simulink model "Vcu"  (R2020a)
settings: Solver=FixedStepDiscrete  StartTime=0.0  StopTime=10.0  FixedStep=ModelSimTime  RelTol=1e-3
PostLoadFcn:
  | , if any(exist('dsrtsu_mdlpostloadfcn', 'file') ~= 0), dsrtsu_mdlpostloadfcn('Execute', bdroot); end,
InitFcn:
  | , if any(exist('rtifpga_mdlclblib', 'file') ~= 0), rtifpga_mdlclblib('Init', bdroot); end,
undefined symbols (not defined in the file): rticanmm_blockfcn, rticanmm_initfcn, sigbuilder_block
libraries: rtimmsu_dsrtlib x5, commutil2 x1
(part 3 of 3)

== system Vcu/Controls /Signal Builder5 ==
  Demux : Demux  Tag=STV Demux  Outputs=1
      settings: DisplayOption=none
  FromWs : FromWorkspace  Tag=STV FromWs  VariableName=tuvar
      SigBuilderData=|
      | common.afterFinalStr = 'Extrapolate'
      | common.sampleTime = 0
      | dataSet.timeRange = [0 10]
      | dataSet.name = 'Group 1'
      | sbobj.Groups.Name = 'Group 1'
      | sbobj.Groups.Signals.Name = 'Driver Button'
      | sbobj.Groups.Signals.XData = [0 6 6 10]
      | sbobj.Groups.Signals.YData = [1 1 2 2]
  Driver Button : Outport  Tag=STV Outport  VectorParamsAs1DForOutWhenUnconnected=off
  wires:
  Demux/1 -> Driver Button/1
  FromWs/1 -> Demux/1

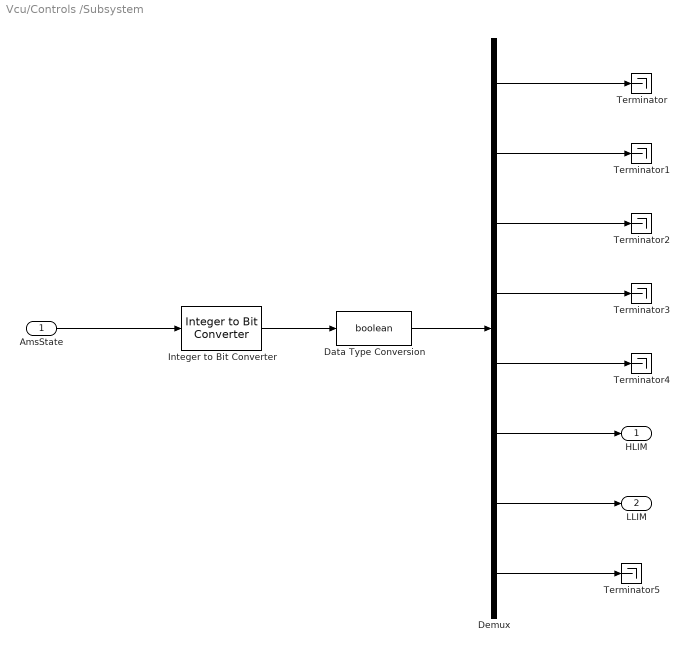
== system Vcu/Controls /Subsystem ==
  AmsState : Inport
  Data Type Conversion : DataTypeConversion  OutDataTypeStr=boolean
  Demux : Demux  Outputs=8
  Integer to Bit Converter : commutil2/Integer to Bit Converter  nbits=8  signedInputValues=Unsigned  bitOrder=LSB first  outDtype=Inherit via internal rule
  Terminator{,1..5} (6 alike) : Terminator
  HLIM : Outport  VectorParamsAs1DForOutWhenUnconnected=off
  LLIM : Outport  Port=2  VectorParamsAs1DForOutWhenUnconnected=off
  wires:
  Integer to Bit Converter/1 -> Data Type Conversion/1
  AmsState/1 -> Integer to Bit Converter/1
  Data Type Conversion/1 -> Demux/1
  Demux/1 -> Terminator/1
  Demux/2 -> Terminator1/1
  Demux/3 -> Terminator2/1
  Demux/4 -> Terminator3/1
  Demux/5 -> Terminator4/1
  Demux/7 -> LLIM/1
  Demux/6 -> HLIM/1
  Demux/8 -> Terminator5/1

== system Vcu/Controls /Triggering2RTICANMM MainBlock ==
  AMK0_ActualValues1 : Subsystem
  AMK0_ActualValues2 : Subsystem
  AMK0_SetPoints1 : Subsystem
  AMK1_ActualValues1 : Subsystem
  AMK1_ActualValues2 : Subsystem
  AMK1_SetPoints1 : Subsystem
  buscreator : BusCreator  Inputs=6
  out : Outport  VectorParamsAs1DForOutWhenUnconnected=off
  wires:
  AMK0_ActualValues1/1(out) -> buscreator/1  "AMK0_ActualValues1"
  AMK0_ActualValues2/1(out) -> buscreator/2  "AMK0_ActualValues2"
  AMK0_SetPoints1/1(out) -> buscreator/3  "AMK0_SetPoints1"
  AMK1_ActualValues1/1(out) -> buscreator/4  "AMK1_ActualValues1"
  AMK1_ActualValues2/1(out) -> buscreator/5  "AMK1_ActualValues2"
  AMK1_SetPoints1/1(out) -> buscreator/6  "AMK1_SetPoints1"
  buscreator/1 -> out/1  "CAN"

== system Vcu/Controls /User2RTICANMM MainBlock ==
  in : Inport
  AMK0_SetPoints1 : Subsystem
  AMK1_SetPoints1 : Subsystem
  buscreator : BusCreator  Inputs=2
  out : Outport  VectorParamsAs1DForOutWhenUnconnected=off
  wires:
  AMK0_SetPoints1/1(out) -> buscreator/1  "AMK0_SetPoints1"
  AMK1_SetPoints1/1(out) -> buscreator/2  "AMK1_SetPoints1"
  in/1 -> AMK0_SetPoints1/1(in), AMK1_SetPoints1/1(in)
  buscreator/1 -> out/1  "CAN"

== system Vcu/Controls /User2RTICANMM MainBlock1 ==
  in : Inport
  AMK0_SetPoints1 : Subsystem
  AMK1_SetPoints1 : Subsystem
  buscreator : BusCreator  Inputs=2
  out : Outport  VectorParamsAs1DForOutWhenUnconnected=off
  wires:
  AMK0_SetPoints1/1(out) -> buscreator/1  "AMK0_SetPoints1"
  AMK1_SetPoints1/1(out) -> buscreator/2  "AMK1_SetPoints1"
  in/1 -> AMK0_SetPoints1/1(in), AMK1_SetPoints1/1(in)
  buscreator/1 -> out/1  "CAN"

== system Vcu/Controls /User2RTICANMM MainBlock2 ==
  CoolingLoopModes : Subsystem
  TemperatureInfo : Subsystem
  VehicleInfo : Subsystem
  buscreator : BusCreator  Inputs=3
  out : Outport  VectorParamsAs1DForOutWhenUnconnected=off
  wires:
  CoolingLoopModes/1(out) -> buscreator/1  "CoolingLoopModes"
  TemperatureInfo/1(out) -> buscreator/2  "TemperatureInfo"
  VehicleInfo/1(out) -> buscreator/3  "VehicleInfo"
  buscreator/1 -> out/1  "CAN"

== system Vcu/Controls /User2RTICANMM MainBlock3 ==
  in : Inport
  ELP_ContactorRequest : Subsystem
  buscreator : BusCreator  Inputs=1
  out : Outport  VectorParamsAs1DForOutWhenUnconnected=off
  wires:
  ELP_ContactorRequest/1(out) -> buscreator/1  "ELP_ContactorRequest"
  in/1 -> ELP_ContactorRequest/1(in)
  buscreator/1 -> out/1  "CAN"

== system Vcu/RTICANMM ControllerSetup/ModelClose ==

== system Vcu/RTICANMM ControllerSetup1/ModelClose ==

== system Vcu/RTICANMM ControllerSetup2/ModelClose ==

== system Vcu/RTICANMM ControllerSetup3/ModelClose ==

== system Vcu/RTICANMM GeneralSetup/ModelClose ==

== system Vcu/Controls /RTICANMM MainBlock/ModelClose ==

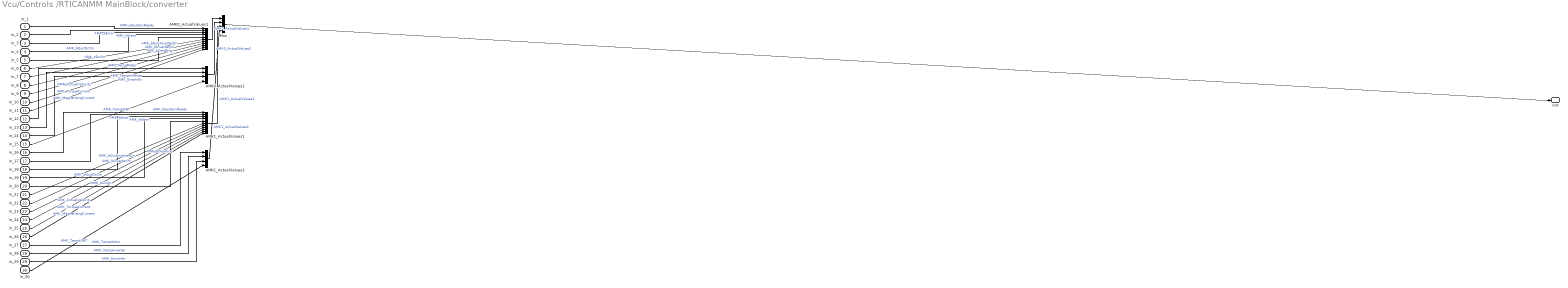
== system Vcu/Controls /RTICANMM MainBlock/converter ==
  in_1 : Inport
  in_2 : Inport  Port=2
  in_3 : Inport  Port=3
  in_4 : Inport  Port=4
  in_5 : Inport  Port=5
  in_6 : Inport  Port=6
  in_7 : Inport  Port=7
  in_8 : Inport  Port=8
  in_9 : Inport  Port=9
  in_10 : Inport  Port=10
  in_11 : Inport  Port=11
  in_12 : Inport  Port=12
  in_13 : Inport  Port=13
  in_14 : Inport  Port=14
  in_15 : Inport  Port=15
  in_16 : Inport  Port=16
  in_17 : Inport  Port=17
  in_18 : Inport  Port=18
  in_19 : Inport  Port=19
  in_20 : Inport  Port=20
  in_21 : Inport  Port=21
  in_22 : Inport  Port=22
  in_23 : Inport  Port=23
  in_24 : Inport  Port=24
  in_25 : Inport  Port=25
  in_26 : Inport  Port=26
  in_27 : Inport  Port=27
  in_28 : Inport  Port=28
  in_29 : Inport  Port=29
  in_30 : Inport  Port=30
  AMK0_ActualValues1 : BusCreator  Inputs=11
  AMK0_ActualValues2 : BusCreator  Inputs=4
  AMK1_ActualValues1 : BusCreator  Inputs=11
  AMK1_ActualValues2 : BusCreator  Inputs=4
  Mux : BusCreator  Inputs=4
  out : Outport
  wires:
  in_1/1 -> AMK0_ActualValues1/1  "AMK_bSystemReady"
  AMK0_ActualValues1/1 -> Mux/1  "AMK0_ActualValues1"
  in_2/1 -> AMK0_ActualValues1/2  "AMK_bError"
  in_3/1 -> AMK0_ActualValues1/3  "AMK_bWarn"
  in_4/1 -> AMK0_ActualValues1/4  "AMK_bQuitDcOn"
  in_5/1 -> AMK0_ActualValues1/5  "AMK_bDcOn"
  in_6/1 -> AMK0_ActualValues1/6  "AMK_bQuitInverterOn"
  in_7/1 -> AMK0_ActualValues1/7  "AMK_bInverterOn"
  in_8/1 -> AMK0_ActualValues1/8  "AMK_bDerating"
  in_9/1 -> AMK0_ActualValues1/9  "AMK_ActualVelocity"
  in_10/1 -> AMK0_ActualValues1/10  "AMK_TorqueCurrent"
  in_11/1 -> AMK0_ActualValues1/11  "AMK_MagnetizingCurrent"
  in_12/1 -> AMK0_ActualValues2/1  "AMK_TempMotor"
  AMK0_ActualValues2/1 -> Mux/2  "AMK0_ActualValues2"
  in_13/1 -> AMK0_ActualValues2/2  "AMK_TempInverter"
  in_14/1 -> AMK0_ActualValues2/3  "AMK_ErrorInfo"
  in_15/1 -> AMK0_ActualValues2/4  "AMK_TempIGBT"
  in_16/1 -> AMK1_ActualValues1/1  "AMK_bSystemReady"
  AMK1_ActualValues1/1 -> Mux/3  "AMK1_ActualValues1"
  in_17/1 -> AMK1_ActualValues1/2  "AMK_bError"
  in_18/1 -> AMK1_ActualValues1/3  "AMK_bWarn"
  in_19/1 -> AMK1_ActualValues1/4  "AMK_bQuitDcOn"
  in_20/1 -> AMK1_ActualValues1/5  "AMK_bDcOn"
  in_21/1 -> AMK1_ActualValues1/6  "AMK_bQuitInverterOn"
  in_22/1 -> AMK1_ActualValues1/7  "AMK_bInverterOn"
  in_23/1 -> AMK1_ActualValues1/8  "AMK_bDerating"
  in_24/1 -> AMK1_ActualValues1/9  "AMK_ActualVelocity"
  in_25/1 -> AMK1_ActualValues1/10  "AMK_TorqueCurrent"
  in_26/1 -> AMK1_ActualValues1/11  "AMK_MagnetizingCurrent"
  in_27/1 -> AMK1_ActualValues2/1  "AMK_TempMotor"
  AMK1_ActualValues2/1 -> Mux/4  "AMK1_ActualValues2"
  in_28/1 -> AMK1_ActualValues2/2  "AMK_TempInverter"
  in_29/1 -> AMK1_ActualValues2/3  "AMK_ErrorInfo"
  in_30/1 -> AMK1_ActualValues2/4  "AMK_TempIGBT"
  Mux/1 -> out/1

== system Vcu/Controls /RTICANMM MainBlock1/ModelClose ==

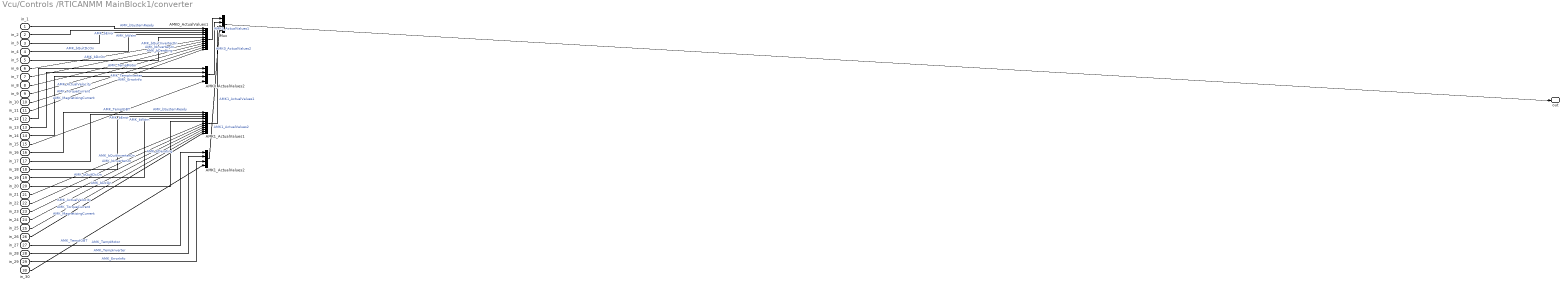
== system Vcu/Controls /RTICANMM MainBlock1/converter ==
  in_1 : Inport
  in_2 : Inport  Port=2
  in_3 : Inport  Port=3
  in_4 : Inport  Port=4
  in_5 : Inport  Port=5
  in_6 : Inport  Port=6
  in_7 : Inport  Port=7
  in_8 : Inport  Port=8
  in_9 : Inport  Port=9
  in_10 : Inport  Port=10
  in_11 : Inport  Port=11
  in_12 : Inport  Port=12
  in_13 : Inport  Port=13
  in_14 : Inport  Port=14
  in_15 : Inport  Port=15
  in_16 : Inport  Port=16
  in_17 : Inport  Port=17
  in_18 : Inport  Port=18
  in_19 : Inport  Port=19
  in_20 : Inport  Port=20
  in_21 : Inport  Port=21
  in_22 : Inport  Port=22
  in_23 : Inport  Port=23
  in_24 : Inport  Port=24
  in_25 : Inport  Port=25
  in_26 : Inport  Port=26
  in_27 : Inport  Port=27
  in_28 : Inport  Port=28
  in_29 : Inport  Port=29
  in_30 : Inport  Port=30
  AMK0_ActualValues1 : BusCreator  Inputs=11
  AMK0_ActualValues2 : BusCreator  Inputs=4
  AMK1_ActualValues1 : BusCreator  Inputs=11
  AMK1_ActualValues2 : BusCreator  Inputs=4
  Mux : BusCreator  Inputs=4
  out : Outport
  wires:
  in_1/1 -> AMK0_ActualValues1/1  "AMK_bSystemReady"
  AMK0_ActualValues1/1 -> Mux/1  "AMK0_ActualValues1"
  in_2/1 -> AMK0_ActualValues1/2  "AMK_bError"
  in_3/1 -> AMK0_ActualValues1/3  "AMK_bWarn"
  in_4/1 -> AMK0_ActualValues1/4  "AMK_bQuitDcOn"
  in_5/1 -> AMK0_ActualValues1/5  "AMK_bDcOn"
  in_6/1 -> AMK0_ActualValues1/6  "AMK_bQuitInverterOn"
  in_7/1 -> AMK0_ActualValues1/7  "AMK_bInverterOn"
  in_8/1 -> AMK0_ActualValues1/8  "AMK_bDerating"
  in_9/1 -> AMK0_ActualValues1/9  "AMK_ActualVelocity"
  in_10/1 -> AMK0_ActualValues1/10  "AMK_TorqueCurrent"
  in_11/1 -> AMK0_ActualValues1/11  "AMK_MagnetizingCurrent"
  in_12/1 -> AMK0_ActualValues2/1  "AMK_TempMotor"
  AMK0_ActualValues2/1 -> Mux/2  "AMK0_ActualValues2"
  in_13/1 -> AMK0_ActualValues2/2  "AMK_TempInverter"
  in_14/1 -> AMK0_ActualValues2/3  "AMK_ErrorInfo"
  in_15/1 -> AMK0_ActualValues2/4  "AMK_TempIGBT"
  in_16/1 -> AMK1_ActualValues1/1  "AMK_bSystemReady"
  AMK1_ActualValues1/1 -> Mux/3  "AMK1_ActualValues1"
  in_17/1 -> AMK1_ActualValues1/2  "AMK_bError"
  in_18/1 -> AMK1_ActualValues1/3  "AMK_bWarn"
  in_19/1 -> AMK1_ActualValues1/4  "AMK_bQuitDcOn"
  in_20/1 -> AMK1_ActualValues1/5  "AMK_bDcOn"
  in_21/1 -> AMK1_ActualValues1/6  "AMK_bQuitInverterOn"
  in_22/1 -> AMK1_ActualValues1/7  "AMK_bInverterOn"
  in_23/1 -> AMK1_ActualValues1/8  "AMK_bDerating"
  in_24/1 -> AMK1_ActualValues1/9  "AMK_ActualVelocity"
  in_25/1 -> AMK1_ActualValues1/10  "AMK_TorqueCurrent"
  in_26/1 -> AMK1_ActualValues1/11  "AMK_MagnetizingCurrent"
  in_27/1 -> AMK1_ActualValues2/1  "AMK_TempMotor"
  AMK1_ActualValues2/1 -> Mux/4  "AMK1_ActualValues2"
  in_28/1 -> AMK1_ActualValues2/2  "AMK_TempInverter"
  in_29/1 -> AMK1_ActualValues2/3  "AMK_ErrorInfo"
  in_30/1 -> AMK1_ActualValues2/4  "AMK_TempIGBT"
  Mux/1 -> out/1

== system Vcu/Controls /RTICANMM MainBlock2/ModelClose ==

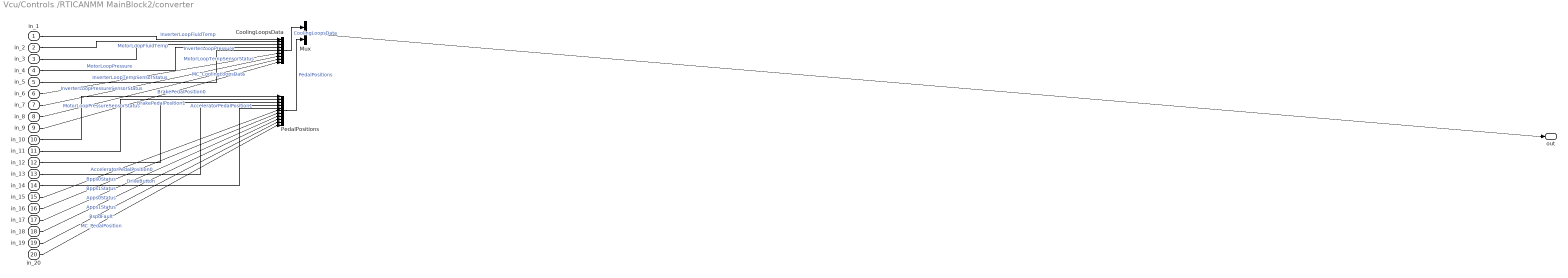
== system Vcu/Controls /RTICANMM MainBlock2/converter ==
  in_1 : Inport
  in_2 : Inport  Port=2
  in_3 : Inport  Port=3
  in_4 : Inport  Port=4
  in_5 : Inport  Port=5
  in_6 : Inport  Port=6
  in_7 : Inport  Port=7
  in_8 : Inport  Port=8
  in_9 : Inport  Port=9
  in_10 : Inport  Port=10
  in_11 : Inport  Port=11
  in_12 : Inport  Port=12
  in_13 : Inport  Port=13
  in_14 : Inport  Port=14
  in_15 : Inport  Port=15
  in_16 : Inport  Port=16
  in_17 : Inport  Port=17
  in_18 : Inport  Port=18
  in_19 : Inport  Port=19
  in_20 : Inport  Port=20
  CoolingLoopsData : BusCreator  Inputs=9
  Mux : BusCreator  Inputs=2
  PedalPositions : BusCreator  Inputs=11
  out : Outport
  wires:
  in_1/1 -> CoolingLoopsData/1  "InverterLoopFluidTemp"
  CoolingLoopsData/1 -> Mux/1  "CoolingLoopsData"
  in_2/1 -> CoolingLoopsData/2  "MotorLoopFluidTemp"
  in_3/1 -> CoolingLoopsData/3  "InverterLoopPressure"
  in_4/1 -> CoolingLoopsData/4  "MotorLoopPressure"
  in_5/1 -> CoolingLoopsData/5  "InverterLoopTempSensorStatus"
  in_6/1 -> CoolingLoopsData/6  "MotorLoopTempSensorStatus"
  in_7/1 -> CoolingLoopsData/7  "InverterLoopPressureSensorStatus"
  in_8/1 -> CoolingLoopsData/8  "MotorLoopPressureSensorStatus"
  in_9/1 -> CoolingLoopsData/9  "MC_CoolingLoopsData"
  in_10/1 -> PedalPositions/1  "BrakePedalPosition0"
  PedalPositions/1 -> Mux/2  "PedalPositions"
  in_11/1 -> PedalPositions/2  "BrakePedalPosition1"
  in_12/1 -> PedalPositions/3  "AcceleratorPedalPosition1"
  in_13/1 -> PedalPositions/4  "AcceleratorPedalPosition0"
  in_14/1 -> PedalPositions/5  "DriveButton"
  in_15/1 -> PedalPositions/6  "Bpps0Status"
  in_16/1 -> PedalPositions/7  "Bpps1Status"
  in_17/1 -> PedalPositions/8  "Apps0Status"
  in_18/1 -> PedalPositions/9  "Apps1Status"
  in_19/1 -> PedalPositions/10  "BspdFault"
  in_20/1 -> PedalPositions/11  "MC_PedalPosition"
  Mux/1 -> out/1

== system Vcu/Controls /RTICANMM MainBlock3/ModelClose ==

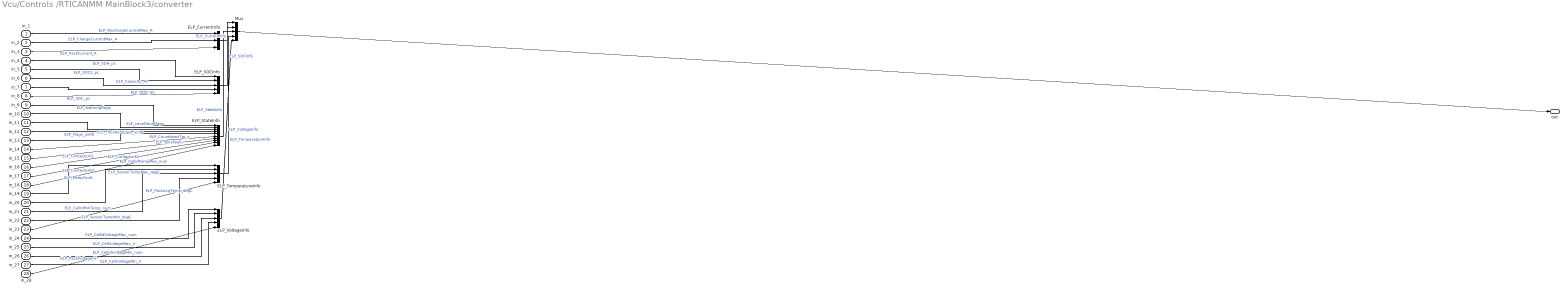
== system Vcu/Controls /RTICANMM MainBlock3/converter ==
  in_1 : Inport
  in_2 : Inport  Port=2
  in_3 : Inport  Port=3
  in_4 : Inport  Port=4
  in_5 : Inport  Port=5
  in_6 : Inport  Port=6
  in_7 : Inport  Port=7
  in_8 : Inport  Port=8
  in_9 : Inport  Port=9
  in_10 : Inport  Port=10
  in_11 : Inport  Port=11
  in_12 : Inport  Port=12
  in_13 : Inport  Port=13
  in_14 : Inport  Port=14
  in_15 : Inport  Port=15
  in_16 : Inport  Port=16
  in_17 : Inport  Port=17
  in_18 : Inport  Port=18
  in_19 : Inport  Port=19
  in_20 : Inport  Port=20
  in_21 : Inport  Port=21
  in_22 : Inport  Port=22
  in_23 : Inport  Port=23
  in_24 : Inport  Port=24
  in_25 : Inport  Port=25
  in_26 : Inport  Port=26
  in_27 : Inport  Port=27
  in_28 : Inport  Port=28
  ELP_CurrentInfo : BusCreator  Inputs=3
  ELP_SOCInfo : BusCreator  Inputs=5
  ELP_StateInfo : BusCreator  Inputs=10
  ELP_TemperatureInfo : BusCreator  Inputs=5
  ELP_VoltageInfo : BusCreator  Inputs=5
  Mux : BusCreator  Inputs=5
  out : Outport
  wires:
  in_1/1 -> ELP_CurrentInfo/1  "ELP_DischargeCurrentMax_A"
  ELP_CurrentInfo/1 -> Mux/1  "ELP_CurrentInfo"
  in_2/1 -> ELP_CurrentInfo/2  "ELP_ChargeCurrentMax_A"
  in_3/1 -> ELP_CurrentInfo/3  "ELP_PackCurrent_A"
  in_4/1 -> ELP_SOCInfo/1  "ELP_SOH_pc"
  ELP_SOCInfo/1 -> Mux/2  "ELP_SOCInfo"
  in_5/1 -> ELP_SOCInfo/2  "ELP_SOC2_pc"
  in_6/1 -> ELP_SOCInfo/3  "ELP_Capacity_Ah"
  in_7/1 -> ELP_SOCInfo/4  "ELP_DOD_Ah"
  in_8/1 -> ELP_SOCInfo/5  "ELP_SOC_pc"
  in_9/1 -> ELP_StateInfo/1  "ELP_WarningFlags"
  ELP_StateInfo/1 -> Mux/3  "ELP_StateInfo"
  in_10/1 -> ELP_StateInfo/2  "ELP_LevelFaultFlags"
  in_11/1 -> ELP_StateInfo/3  "ELP_FltCodeStored_uint8"
  in_12/1 -> ELP_StateInfo/4  "ELP_Flags_uint8"
  in_13/1 -> ELP_StateInfo/5  "ELP_CountdownTm_s"
  in_14/1 -> ELP_StateInfo/6  "ELP_BmsFault"
  in_15/1 -> ELP_StateInfo/7  "ELP_ContactorK1"
  in_16/1 -> ELP_StateInfo/8  "ELP_ContactorK2"
  in_17/1 -> ELP_StateInfo/9  "ELP_ContactorK3"
  in_18/1 -> ELP_StateInfo/10  "ELP_RelayFault"
  in_19/1 -> ELP_TemperatureInfo/1  "ELP_CellIdTempMax_num"
  ELP_TemperatureInfo/1 -> Mux/4  "ELP_TemperatureInfo"
  in_20/1 -> ELP_TemperatureInfo/2  "ELP_SensorTempMax_degC"
  in_21/1 -> ELP_TemperatureInfo/3  "ELP_CellIdMinTemp_num"
  in_22/1 -> ELP_TemperatureInfo/4  "ELP_SensorTempMin_degC"
  in_23/1 -> ELP_TemperatureInfo/5  "ELP_PackAvgTemp_degC"
  in_24/1 -> ELP_VoltageInfo/1  "ELP_CellIdVoltageMax_num"
  ELP_VoltageInfo/1 -> Mux/5  "ELP_VoltageInfo"
  in_25/1 -> ELP_VoltageInfo/2  "ELP_CellVoltageMax_V"
  in_26/1 -> ELP_VoltageInfo/3  "ELP_CellIdVoltageMin_num"
  in_27/1 -> ELP_VoltageInfo/4  "ELP_CellVoltageMin_V"
  in_28/1 -> ELP_VoltageInfo/5  "ELP_PackVoltage_V"
  Mux/1 -> out/1

== system Vcu/Controls /Triggering2RTICANMM MainBlock/AMK0_ActualValues1 ==
  AMK0_ActualValues1_CycleTime : Constant  Value=0
  buscreator : BusCreator  Inputs=1
  dt_AMK0_ActualValues1_CycleTime : DataTypeConversion  RndMeth=Zero
  out : Outport
  wires:
  buscreator/1 -> out/1  "AMK0_ActualValues1"
  AMK0_ActualValues1_CycleTime/1 -> dt_AMK0_ActualValues1_CycleTime/1
  dt_AMK0_ActualValues1_CycleTime/1 -> buscreator/1  "AMK0_ActualValues1_CycleTime"

== system Vcu/Controls /Triggering2RTICANMM MainBlock/AMK0_ActualValues2 ==
  AMK0_ActualValues2_CycleTime : Constant  Value=0
  buscreator : BusCreator  Inputs=1
  dt_AMK0_ActualValues2_CycleTime : DataTypeConversion  RndMeth=Zero
  out : Outport
  wires:
  buscreator/1 -> out/1  "AMK0_ActualValues2"
  AMK0_ActualValues2_CycleTime/1 -> dt_AMK0_ActualValues2_CycleTime/1
  dt_AMK0_ActualValues2_CycleTime/1 -> buscreator/1  "AMK0_ActualValues2_CycleTime"

== system Vcu/Controls /Triggering2RTICANMM MainBlock/AMK0_SetPoints1 ==
  AMK0_SetPoints1_CycleTime : Constant  Value=0
  buscreator : BusCreator  Inputs=1
  dt_AMK0_SetPoints1_CycleTime : DataTypeConversion  RndMeth=Zero
  out : Outport
  wires:
  buscreator/1 -> out/1  "AMK0_SetPoints1"
  AMK0_SetPoints1_CycleTime/1 -> dt_AMK0_SetPoints1_CycleTime/1
  dt_AMK0_SetPoints1_CycleTime/1 -> buscreator/1  "AMK0_SetPoints1_CycleTime"

== system Vcu/Controls /Triggering2RTICANMM MainBlock/AMK1_ActualValues1 ==
  AMK1_ActualValues1_CycleTime : Constant  Value=0
  buscreator : BusCreator  Inputs=1
  dt_AMK1_ActualValues1_CycleTime : DataTypeConversion  RndMeth=Zero
  out : Outport
  wires:
  buscreator/1 -> out/1  "AMK1_ActualValues1"
  AMK1_ActualValues1_CycleTime/1 -> dt_AMK1_ActualValues1_CycleTime/1
  dt_AMK1_ActualValues1_CycleTime/1 -> buscreator/1  "AMK1_ActualValues1_CycleTime"

== system Vcu/Controls /Triggering2RTICANMM MainBlock/AMK1_ActualValues2 ==
  AMK1_ActualValues2_CycleTime : Constant  Value=0
  buscreator : BusCreator  Inputs=1
  dt_AMK1_ActualValues2_CycleTime : DataTypeConversion  RndMeth=Zero
  out : Outport
  wires:
  buscreator/1 -> out/1  "AMK1_ActualValues2"
  AMK1_ActualValues2_CycleTime/1 -> dt_AMK1_ActualValues2_CycleTime/1
  dt_AMK1_ActualValues2_CycleTime/1 -> buscreator/1  "AMK1_ActualValues2_CycleTime"

== system Vcu/Controls /Triggering2RTICANMM MainBlock/AMK1_SetPoints1 ==
  AMK1_SetPoints1_CycleTime : Constant  Value=0
  buscreator : BusCreator  Inputs=1
  dt_AMK1_SetPoints1_CycleTime : DataTypeConversion  RndMeth=Zero
  out : Outport
  wires:
  buscreator/1 -> out/1  "AMK1_SetPoints1"
  AMK1_SetPoints1_CycleTime/1 -> dt_AMK1_SetPoints1_CycleTime/1
  dt_AMK1_SetPoints1_CycleTime/1 -> buscreator/1  "AMK1_SetPoints1_CycleTime"

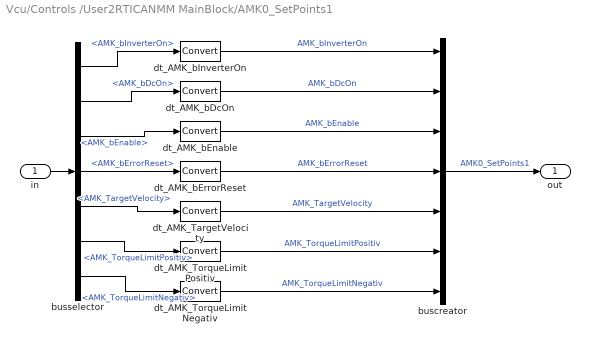
== system Vcu/Controls /User2RTICANMM MainBlock/AMK0_SetPoints1 ==
  in : Inport
  buscreator : BusCreator  Inputs=7
  busselector : BusSelector  OutputSignals=Inverter1FL.AMK_bInverterOn,Inverter1FL.AMK_bDcOn,Inverter1FL.AMK_bEnable,Inverter1FL.AMK_bErrorReset,Inverter1FL.AMK_TargetVelocity,Inverter1FL.AMK_TorqueLimitPositiv,Inverter1FL.AMK_TorqueLimitNegativ
  dt_AMK_TargetVelocity : DataTypeConversion  RndMeth=Zero
  dt_AMK_TorqueLimitNegativ : DataTypeConversion  RndMeth=Zero
  dt_AMK_TorqueLimitPositiv : DataTypeConversion  RndMeth=Zero
  dt_AMK_bDcOn : DataTypeConversion  RndMeth=Zero
  dt_AMK_bEnable : DataTypeConversion  RndMeth=Zero
  dt_AMK_bErrorReset : DataTypeConversion  RndMeth=Zero
  dt_AMK_bInverterOn : DataTypeConversion  RndMeth=Zero
  out : Outport
  wires:
  buscreator/1 -> out/1  "AMK0_SetPoints1"
  in/1 -> busselector/1
  busselector/1 -> dt_AMK_bInverterOn/1  "<AMK_bInverterOn>"
  dt_AMK_bInverterOn/1 -> buscreator/1  "AMK_bInverterOn"
  busselector/2 -> dt_AMK_bDcOn/1  "<AMK_bDcOn>"
  dt_AMK_bDcOn/1 -> buscreator/2  "AMK_bDcOn"
  busselector/3 -> dt_AMK_bEnable/1  "<AMK_bEnable>"
  dt_AMK_bEnable/1 -> buscreator/3  "AMK_bEnable"
  busselector/4 -> dt_AMK_bErrorReset/1  "<AMK_bErrorReset>"
  dt_AMK_bErrorReset/1 -> buscreator/4  "AMK_bErrorReset"
  busselector/5 -> dt_AMK_TargetVelocity/1  "<AMK_TargetVelocity>"
  dt_AMK_TargetVelocity/1 -> buscreator/5  "AMK_TargetVelocity"
  busselector/6 -> dt_AMK_TorqueLimitPositiv/1  "<AMK_TorqueLimitPositiv>"
  dt_AMK_TorqueLimitPositiv/1 -> buscreator/6  "AMK_TorqueLimitPositiv"
  busselector/7 -> dt_AMK_TorqueLimitNegativ/1  "<AMK_TorqueLimitNegativ>"
  dt_AMK_TorqueLimitNegativ/1 -> buscreator/7  "AMK_TorqueLimitNegativ"

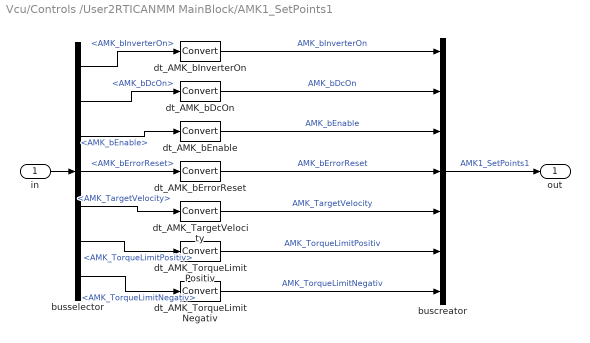
== system Vcu/Controls /User2RTICANMM MainBlock/AMK1_SetPoints1 ==
  in : Inport
  buscreator : BusCreator  Inputs=7
  busselector : BusSelector  OutputSignals=Inverter2FR.AMK_bInverterOn,Inverter2FR.AMK_bDcOn,Inverter2FR.AMK_bEnable,Inverter2FR.AMK_bErrorReset,Inverter2FR.AMK_TargetVelocity,Inverter2FR.AMK_TorqueLimitPositiv,Inverter2FR.AMK_TorqueLimitNegativ
  dt_AMK_TargetVelocity : DataTypeConversion  RndMeth=Zero
  dt_AMK_TorqueLimitNegativ : DataTypeConversion  RndMeth=Zero
  dt_AMK_TorqueLimitPositiv : DataTypeConversion  RndMeth=Zero
  dt_AMK_bDcOn : DataTypeConversion  RndMeth=Zero
  dt_AMK_bEnable : DataTypeConversion  RndMeth=Zero
  dt_AMK_bErrorReset : DataTypeConversion  RndMeth=Zero
  dt_AMK_bInverterOn : DataTypeConversion  RndMeth=Zero
  out : Outport
  wires:
  buscreator/1 -> out/1  "AMK1_SetPoints1"
  in/1 -> busselector/1
  busselector/1 -> dt_AMK_bInverterOn/1  "<AMK_bInverterOn>"
  dt_AMK_bInverterOn/1 -> buscreator/1  "AMK_bInverterOn"
  busselector/2 -> dt_AMK_bDcOn/1  "<AMK_bDcOn>"
  dt_AMK_bDcOn/1 -> buscreator/2  "AMK_bDcOn"
  busselector/3 -> dt_AMK_bEnable/1  "<AMK_bEnable>"
  dt_AMK_bEnable/1 -> buscreator/3  "AMK_bEnable"
  busselector/4 -> dt_AMK_bErrorReset/1  "<AMK_bErrorReset>"
  dt_AMK_bErrorReset/1 -> buscreator/4  "AMK_bErrorReset"
  busselector/5 -> dt_AMK_TargetVelocity/1  "<AMK_TargetVelocity>"
  dt_AMK_TargetVelocity/1 -> buscreator/5  "AMK_TargetVelocity"
  busselector/6 -> dt_AMK_TorqueLimitPositiv/1  "<AMK_TorqueLimitPositiv>"
  dt_AMK_TorqueLimitPositiv/1 -> buscreator/6  "AMK_TorqueLimitPositiv"
  busselector/7 -> dt_AMK_TorqueLimitNegativ/1  "<AMK_TorqueLimitNegativ>"
  dt_AMK_TorqueLimitNegativ/1 -> buscreator/7  "AMK_TorqueLimitNegativ"

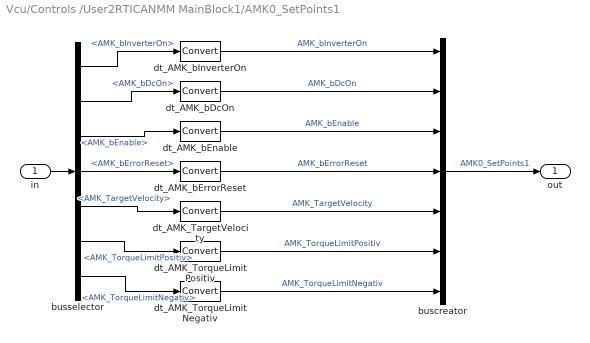
== system Vcu/Controls /User2RTICANMM MainBlock1/AMK0_SetPoints1 ==
  in : Inport
  buscreator : BusCreator  Inputs=7
  busselector : BusSelector  OutputSignals=Inverter3RL.AMK_bInverterOn,Inverter3RL.AMK_bDcOn,Inverter3RL.AMK_bEnable,Inverter3RL.AMK_bErrorReset,Inverter3RL.AMK_TargetVelocity,Inverter3RL.AMK_TorqueLimitPositiv,Inverter3RL.AMK_TorqueLimitNegativ
  dt_AMK_TargetVelocity : DataTypeConversion  RndMeth=Zero
  dt_AMK_TorqueLimitNegativ : DataTypeConversion  RndMeth=Zero
  dt_AMK_TorqueLimitPositiv : DataTypeConversion  RndMeth=Zero
  dt_AMK_bDcOn : DataTypeConversion  RndMeth=Zero
  dt_AMK_bEnable : DataTypeConversion  RndMeth=Zero
  dt_AMK_bErrorReset : DataTypeConversion  RndMeth=Zero
  dt_AMK_bInverterOn : DataTypeConversion  RndMeth=Zero
  out : Outport
  wires:
  buscreator/1 -> out/1  "AMK0_SetPoints1"
  in/1 -> busselector/1
  busselector/1 -> dt_AMK_bInverterOn/1  "<AMK_bInverterOn>"
  dt_AMK_bInverterOn/1 -> buscreator/1  "AMK_bInverterOn"
  busselector/2 -> dt_AMK_bDcOn/1  "<AMK_bDcOn>"
  dt_AMK_bDcOn/1 -> buscreator/2  "AMK_bDcOn"
  busselector/3 -> dt_AMK_bEnable/1  "<AMK_bEnable>"
  dt_AMK_bEnable/1 -> buscreator/3  "AMK_bEnable"
  busselector/4 -> dt_AMK_bErrorReset/1  "<AMK_bErrorReset>"
  dt_AMK_bErrorReset/1 -> buscreator/4  "AMK_bErrorReset"
  busselector/5 -> dt_AMK_TargetVelocity/1  "<AMK_TargetVelocity>"
  dt_AMK_TargetVelocity/1 -> buscreator/5  "AMK_TargetVelocity"
  busselector/6 -> dt_AMK_TorqueLimitPositiv/1  "<AMK_TorqueLimitPositiv>"
  dt_AMK_TorqueLimitPositiv/1 -> buscreator/6  "AMK_TorqueLimitPositiv"
  busselector/7 -> dt_AMK_TorqueLimitNegativ/1  "<AMK_TorqueLimitNegativ>"
  dt_AMK_TorqueLimitNegativ/1 -> buscreator/7  "AMK_TorqueLimitNegativ"

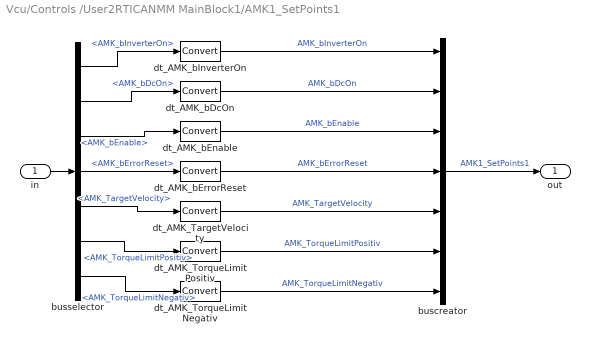
== system Vcu/Controls /User2RTICANMM MainBlock1/AMK1_SetPoints1 ==
  in : Inport
  buscreator : BusCreator  Inputs=7
  busselector : BusSelector  OutputSignals=Inverter4RR.AMK_bInverterOn,Inverter4RR.AMK_bDcOn,Inverter4RR.AMK_bEnable,Inverter4RR.AMK_bErrorReset,Inverter4RR.AMK_TargetVelocity,Inverter4RR.AMK_TorqueLimitPositiv,Inverter4RR.AMK_TorqueLimitNegativ
  dt_AMK_TargetVelocity : DataTypeConversion  RndMeth=Zero
  dt_AMK_TorqueLimitNegativ : DataTypeConversion  RndMeth=Zero
  dt_AMK_TorqueLimitPositiv : DataTypeConversion  RndMeth=Zero
  dt_AMK_bDcOn : DataTypeConversion  RndMeth=Zero
  dt_AMK_bEnable : DataTypeConversion  RndMeth=Zero
  dt_AMK_bErrorReset : DataTypeConversion  RndMeth=Zero
  dt_AMK_bInverterOn : DataTypeConversion  RndMeth=Zero
  out : Outport
  wires:
  buscreator/1 -> out/1  "AMK1_SetPoints1"
  in/1 -> busselector/1
  busselector/1 -> dt_AMK_bInverterOn/1  "<AMK_bInverterOn>"
  dt_AMK_bInverterOn/1 -> buscreator/1  "AMK_bInverterOn"
  busselector/2 -> dt_AMK_bDcOn/1  "<AMK_bDcOn>"
  dt_AMK_bDcOn/1 -> buscreator/2  "AMK_bDcOn"
  busselector/3 -> dt_AMK_bEnable/1  "<AMK_bEnable>"
  dt_AMK_bEnable/1 -> buscreator/3  "AMK_bEnable"
  busselector/4 -> dt_AMK_bErrorReset/1  "<AMK_bErrorReset>"
  dt_AMK_bErrorReset/1 -> buscreator/4  "AMK_bErrorReset"
  busselector/5 -> dt_AMK_TargetVelocity/1  "<AMK_TargetVelocity>"
  dt_AMK_TargetVelocity/1 -> buscreator/5  "AMK_TargetVelocity"
  busselector/6 -> dt_AMK_TorqueLimitPositiv/1  "<AMK_TorqueLimitPositiv>"
  dt_AMK_TorqueLimitPositiv/1 -> buscreator/6  "AMK_TorqueLimitPositiv"
  busselector/7 -> dt_AMK_TorqueLimitNegativ/1  "<AMK_TorqueLimitNegativ>"
  dt_AMK_TorqueLimitNegativ/1 -> buscreator/7  "AMK_TorqueLimitNegativ"

== system Vcu/Controls /User2RTICANMM MainBlock2/CoolingLoopModes ==
  InverterLoopFanMode : Ground
  InverterLoopPumpMode : Ground
  MotorLoopFanMode : Ground
  MotorLoopPumpMode : Ground
  SpeakerRequest : Ground
  buscreator : BusCreator  Inputs=5
  out : Outport
  wires:
  buscreator/1 -> out/1  "CoolingLoopModes"
  InverterLoopFanMode/1 -> buscreator/1  "InverterLoopFanMode"
  InverterLoopPumpMode/1 -> buscreator/2  "InverterLoopPumpMode"
  SpeakerRequest/1 -> buscreator/3  "SpeakerRequest"
  MotorLoopFanMode/1 -> buscreator/4  "MotorLoopFanMode"
  MotorLoopPumpMode/1 -> buscreator/5  "MotorLoopPumpMode"

== system Vcu/Controls /User2RTICANMM MainBlock2/TemperatureInfo ==
  BatteryTemperature : Ground
  LeftFrontMotorTemperature : Ground
  LeftRearMotorTemperature : Ground
  RightFrontMotorTemperature : Ground
  RightRearMotorTemperature : Ground
  buscreator : BusCreator  Inputs=5
  out : Outport
  wires:
  buscreator/1 -> out/1  "TemperatureInfo"
  LeftFrontMotorTemperature/1 -> buscreator/1  "LeftFrontMotorTemperature"
  LeftRearMotorTemperature/1 -> buscreator/2  "LeftRearMotorTemperature"
  RightFrontMotorTemperature/1 -> buscreator/3  "RightFrontMotorTemperature"
  RightRearMotorTemperature/1 -> buscreator/4  "RightRearMotorTemperature"
  BatteryTemperature/1 -> buscreator/5  "BatteryTemperature"

== system Vcu/Controls /User2RTICANMM MainBlock2/VehicleInfo ==
  MaximumPowerAvailablePercentage : Ground
  SocPercentage : Ground
  VcuErrors : Ground
  VehicleSpeed : Ground
  VehicleStatus : Ground
  buscreator : BusCreator  Inputs=5
  out : Outport
  wires:
  buscreator/1 -> out/1  "VehicleInfo"
  MaximumPowerAvailablePercentage/1 -> buscreator/1  "MaximumPowerAvailablePercentage"
  SocPercentage/1 -> buscreator/2  "SocPercentage"
  VcuErrors/1 -> buscreator/3  "VcuErrors"
  VehicleSpeed/1 -> buscreator/4  "VehicleSpeed"
  VehicleStatus/1 -> buscreator/5  "VehicleStatus"

== system Vcu/Controls /User2RTICANMM MainBlock3/ELP_ContactorRequest ==
  in : Inport
  buscreator : BusCreator  Inputs=1
  busselector : BusSelector  OutputSignals=contactor
  dt_ELP_Contactor : DataTypeConversion  RndMeth=Zero
  out : Outport
  wires:
  buscreator/1 -> out/1  "ELP_ContactorRequest"
  in/1 -> busselector/1
  busselector/1 -> dt_ELP_Contactor/1  "<contactor>"
  dt_ELP_Contactor/1 -> buscreator/1  "ELP_Contactor"
